simulink model "model"  (R2019b)
settings: Solver=VariableStepAuto  StartTime=0.0  StopTime=sim_time  FixedStep=Ts/100  RelTol=1e-3
StopFcn:
  | %figure;plot(true_position.Data(:,1),true_position.Data(:,2))
  | 
  | figure;hold on;
  | plot(ref_pos.Data(:,1),ref_pos.Data(:,2));
  | plot(ref_pos_noLA.Data(:,1),ref_pos_noLA.Data(:,2));
  | plot(meas_pos.Data(:,1),meas_pos.Data(:,2));
  | title('Position');
  | xlabel('x (m)');
  | ylabel('y (m)');
  | legend('Reference Position','Reference Position without Look-Ahead','Measured Position');
values from neighbouring files (symbols this model uses):
  b = 1.095    [main.m]
  bike_params = [g h b a lambda m]    [main.m]
  complementary = 0.985    [main.m]
  D_balancing = 0.05    [main.m]
  D_heading = 0    [main.m]
  D_lateral = -0.0    (= 0)    [main.m]
  D_steering_position = 0    [main.m]
  g = 9.81    [main.m]
  g1_den = [1]    [main.m]
  g1_num = 3*[1]    [main.m]
  g2_den = [1]    [main.m]
  g2_num = 5*[1]    [main.m]
  heading_control = 1    [main.m]
  I_balancing = 0    [main.m]
  I_heading = 0    [main.m]
  I_lateral = -0.1    [main.m]
  I_steering_position = 30    [main.m]
  IMU_height = 0.45    [main.m]
  initial_roll = deg2rad(0)    [main.m]
  initial_rollrate = deg2rad(0)    [main.m]
  initial_x = 0    [main.m]
  initial_y = 0    [main.m]
  lambda = deg2rad(70)    [main.m]
  lateral_control = 1    [main.m]
  look_ahead = 0    [main.m]
  look_ahead_time = 2.0    (= 2)    [main.m]
  num_tf_steering = [253.4]    [main.m]
  P_balancing = 1    [main.m]
  P_heading = 0.1    [main.m]
  P_lateral = -0.1    [main.m]
  P_steering_position = 30    [main.m]
  path_tracking = 1    [main.m]
  path_x = path_x'    [paths.m]
  path_y = movmean(path_y,200)    [paths.m]
  roll_rate_coef = 0.9    [main.m]
  time_balance = 10    [main.m]
  Ts = 0.01    [main.m]
  v = 4    [main.m]
undefined symbols (not defined in the file or in its folder): A, B, C, cumulative_dist_along_path, curvature, D, den_filt_steeringrate, DiscIntNeverNeededParam, num_filt_steeringrate, Ts_IMU
libraries: simulink_extras x7, simulink x6, dspsigops x3, cstblocks x1
(part 2 of 2)

== system model/Physical Bike/Global Angles and Coordinates Calculator - Position/Measured Global Angles to Global Coordinates ==
  Velocity : Inport
  Psi : Inport  Port=2
  Beta : Inport  Port=3
  Integrator1 : Integrator
  Integrator2 : Integrator
  MATLAB Function1 : MATLAB Function  TreatAsAtomicUnit=on
  Mux : Mux  Inputs=2
  "Position (X, Y)" : Outport  VectorParamsAs1DForOutWhenUnconnected=off
  wires:
  MATLAB Function1/2(Ydot) -> Integrator2/1  "Ydot"
  MATLAB Function1/1(Xdot) -> Integrator1/1  "Xdot"
  Psi/1 -> MATLAB Function1/2(psi)
  Beta/1 -> MATLAB Function1/3(beta)
  Velocity/1 -> MATLAB Function1/1(v)
  Integrator2/1 -> Mux/2
  Integrator1/1 -> Mux/1
  Mux/1 -> "Position (X, Y)"/1

== system model/IMU + Complementary Filter/Complementary filter/Roll Angle Estimation of Accelerometer/Centripetal Acceleration Compensator ==
  Steering Angle : Inport
  Velocity : Inport  Port=2
  Bike Model b : Constant  Value=b
  Divide : Product  Inputs=*/
  Gain : Gain  Gain=sin(lambda)
  Multiply : Product
  Square : Math  Operator=square  SaturateOnIntegerOverflow=on
  Tan : Trigonometry  Operator=tan
  Estimated Centripetal Acceleration : Outport  VectorParamsAs1DForOutWhenUnconnected=off
  wires:
  Velocity/1 -> Square/1
  Square/1 -> Divide/1
  Bike Model b/1 -> Divide/2
  Steering Angle/1 -> Gain/1
  Divide/1 -> Multiply/1
  Tan/1 -> Multiply/2
  Multiply/1 -> Estimated Centripetal Acceleration/1
  Gain/1 -> Tan/1

== system model/IMU + Complementary Filter/Complementary filter/Roll Angle Estimation of Accelerometer/Lateral Acceleration Compensator ==
  Roll Rate : Inport
  Constant4 : Constant  Value=IMU_height
  Low Pass Filter : Subsystem
  Multiply1 : Product
  Numerical Derivative : Subsystem
  Estimated Lateral Accelerattion due to Roll : Outport  VectorParamsAs1DForOutWhenUnconnected=off
  wires:
  Roll Rate/1 -> Low Pass Filter/1(Roll Rate)
  Constant4/1 -> Multiply1/1
  Multiply1/1 -> Estimated Lateral Accelerattion due to Roll/1  "lateral acceleration"
  Low Pass Filter/1(Filtered Roll Rate) -> Numerical Derivative/1(Roll Rate)
  Numerical Derivative/1(Roll Acceleration) -> Multiply1/2

== system model/IMU + Complementary Filter/Complementary filter/Roll Angle Estimation of Accelerometer/Lateral Acceleration Compensator/Low Pass Filter ==
  Roll Rate : Inport
  Delay18 : Delay  DelayLength=1
  Gain4 : Gain  Gain=roll_rate_coef
  Gain6 : Gain  Gain=1-roll_rate_coef
  Sum4 : Sum  Inputs=|++
  Filtered Roll Rate : Outport  VectorParamsAs1DForOutWhenUnconnected=off
  wires:
  Gain6/1 -> Sum4/1
  Gain4/1 -> Sum4/2
  Sum4/1 -> Filtered Roll Rate/1, Delay18/1  "Filtered Roll Rate"
  Delay18/1 -> Gain4/1
  Roll Rate/1 -> Gain6/1  "Measured Roll Rate"

== system model/IMU + Complementary Filter/Complementary filter/Roll Angle Estimation of Accelerometer/Lateral Acceleration Compensator/Numerical Derivative ==
  Roll Rate : Inport
  Delay18 : Delay  DelayLength=1
  Gain3 : Gain  Gain=1/Ts
  Sum3 : Sum  Inputs=|+-
  Roll Acceleration : Outport  VectorParamsAs1DForOutWhenUnconnected=off
  wires:
  Sum3/1 -> Gain3/1
  Delay18/1 -> Sum3/2
  Roll Rate/1 -> Sum3/1, Delay18/1
  Gain3/1 -> Roll Acceleration/1

== matlab function model/Reference Position/Variable Look Ahead/Look-Ahead Coefficient Selector ==
  data: curv_next input; look_ahead output; curv input
function look_ahead = fcn(curv_next, curv)


if curv>-0.01 && curv<0.01
    curv=0;
end

if curv_next>-0.01 && curv_next<0.01
    curv_next=0;
end



if curv>=0
    if curv-curv_next>0
        look_ahead=0;
    else
        look_ahead=curv_next-curv;
    end
else
    if curv-curv_next<0
        look_ahead=0;
    else
        look_ahead=curv-curv_next;
    end
end



end

== matlab function model/Global Angles and Coordinates Calculator - Position/Measured Bike Angles to Global Angles/MATLAB Function ==
  data: v input; parameters_model input; delta input; psi_d output; beta output
function [psi_d, beta]  = fcn(v, parameters_model, delta)

b = parameters_model(3);
a = parameters_model(4);

beta = ((a / (b)) * (delta));
psi_d = (v / a) * (beta);

% beta = atan((a / (b)) * tan(delta));
% psi_d = (v / a) * sin(beta);

== matlab function model/Reference Position/Variable Look Ahead/Look-Ahead Coefficient Modifier (Slow Turn-Off)  ==
  data: look_ahead input; look_ahead_modified output; feedback input; time input; time_delayed input
function look_ahead_modified = fcn(look_ahead, feedback, time, time_delayed)
% If the look_ahead distance at the current time step is smaller than
% the previous one minues 0.0001 (it got reduced by 'too much')
% then we instead reduced it by a smaller value 'delta' such that
% the look_ahead vanishes in a time kill_time

step=time-time_delayed;

kill_time=3;

delta=(feedback*step)/kill_time;

if look_ahead-feedback<-0.0001
    look_ahead_modified=feedback-delta;
else
    look_ahead_modified = look_ahead;
end
    

end

== matlab function model/Global Angles and Coordinates Calculator - Position/Measured Global Angles to Global Coordinates/MATLAB Function1 ==
  data: v input; psi input; Xdot output; beta input; Ydot output
function [Xdot, Ydot]  = fcn(v, psi, beta)

Xdot = v * cos(psi + beta);
Ydot = v * sin(psi + beta);

== matlab function model/Physical Bike/Global Angles and Coordinates Calculator - Position/Measured Bike Angles to Global Angles/MATLAB Function ==
  data: v input; bike_params input; delta input; psi_d output; beta output
function [psi_d, beta]  = fcn(v, bike_params, delta)

b = bike_params(3);
a = bike_params(4);

beta = atan((a / (b)) * tan(delta));
psi_d = (v / a) * sin(beta);

== matlab function model/Physical Bike/Global Angles and Coordinates Calculator - Position/Measured Global Angles to Global Coordinates/MATLAB Function1 ==
  data: v input; psi input; Xdot output; beta input; Ydot output
function [Xdot, Ydot]  = fcn(v, psi, beta)

Xdot = v * cos(psi + beta);
Ydot = v * sin(psi + beta);
